simulink model "Test"  (R2018a)
settings: Solver=VariableStepAuto  StartTime=0.0  StopTime=1  RelTol=1e-3
libraries: powerlib x37, dspstat3 x1
settings Model: Creator=AL-MOSTAFA  LastModifiedBy=AL-MOSTAFA

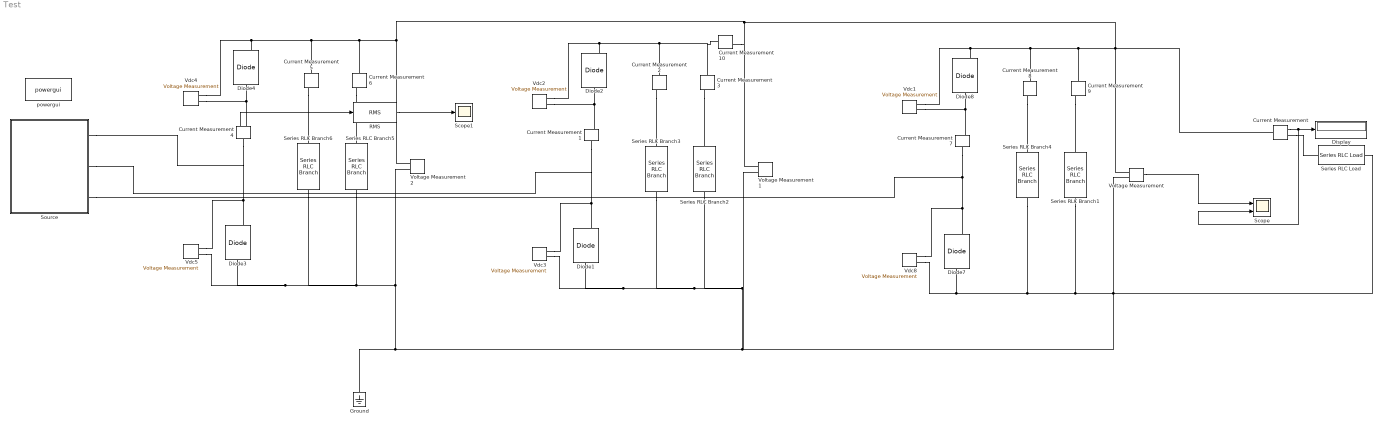
== system Test ==
  Current Measurement{,1..9} (10 alike) : powerlib/Measurements/Current Measurement  PhasorSimulation=off  OutputType=Complex  PSBequivalent=0
  Current Measurement10 : powerlib/Measurements/Current Measurement  PhasorSimulation=off  OutputType=Magnitude  PSBequivalent=0
  Diode{1..4,7..8} (6 alike) : powerlib/Power Electronics/Diode  Ron=0.001  Lon=0  Vf=0.8  IC=0  UseSnubber=0  Rs=500  Cs=250e-9  Measurements=on
  Display : Display
  Ground : powerlib/Elements/Ground  LConnTagsString=a
  RMS : dspstat3/RMS  run=off  directionMode=Each column  dimension=1  InputProcessing=Columns as channels (frame based)  reset_popup=None
  Scope : Scope  NumInputPorts=2
  Scope1 : Scope
  Series RLC Branch{1..6} (6 alike) : powerlib/Elements/Series RLC Branch  LConnTagsString=__new0  RConnTagsString=__new0  BranchType=C  Resistance=10  Inductance=1e-3  SetiL0=off  InitialCurrent=0  Capacitance=500*10^-6  Setx0=off  InitialVoltage=0  Measurements=None
  Series RLC Load : powerlib/Elements/Series RLC Load  LConnTagsString=a  RConnTagsString=__new0  NominalVoltage=500  NominalFrequency=60  ActivePower=5e3  InductivePower=0  CapacitivePower=0  Setx0=off  InitialVoltage=0  SetiL0=off  InitialCurrent=0  Measurements=None  LoadType=constant Z
  Source : Subsystem
  Vdc{1..5,8} (6 alike) : powerlib/Measurements/Voltage Measurement  PhasorSimulation=off  OutputType=Complex  PSBequivalent=0
  Voltage Measurement : powerlib/Measurements/Voltage Measurement  PhasorSimulation=off  OutputType=Complex  PSBequivalent=0
  Voltage Measurement1 : powerlib/Measurements/Voltage Measurement  PhasorSimulation=off  OutputType=Complex  PSBequivalent=0
  Voltage Measurement2 : powerlib/Measurements/Voltage Measurement  PhasorSimulation=off  OutputType=Complex  PSBequivalent=0
  powergui : powerlib/powergui  Priority=1  SimulationMode=Continuous  SampleTime=50e-6  frequency=60  Iterations=50  frequencyindice=50  Pbase=100e6  ErrMax=1e-4  UnitsV=kV  UnitsW=MW  buscounter=0  FunctionMessages=off  echomessages=off  EnableUseOfTLC=off  CurrentSourceSwitches=off  DisableSnubberDevices=off  DisableRonSwitches=off  DisableVfSwitches=off  DisplayEquations=off  SolverType=Tustin/Backward Euler (TBE)  Interpol=off  ExternalGateDelay=off  methode=off  Ts=100  x0status=blocks  SPID=on  SwTol=0  HookPort=off  RestoreLinks=warning  ResistiveCurrentMeasurement=off  Frange=[0:2:500]  Ylog=off  Xlog=on  ShowGrid=off  save=off  variable=ZData  structure=0  ZoomFFT=off  StartTime=0.0  cycles=1  DisplayStyle=1  fundamental=60  FreqAxis=off  MaxFrequency=1000  frequencyindicesteady=1  RmsSteady=1  display=off
  wires:
  Current Measurement/1 -> Scope/2, Display/1
  Current Measurement4/1 -> RMS/1
  Voltage Measurement/1 -> Scope/1
  RMS/1 -> Scope1/1
  connections:
  Current Measurement/RConn1 -- Series RLC Load/LConn1
  Current Measurement7/RConn1 -- Diode8/LConn1 -- Vdc1/LConn1
  Series RLC Branch1/RConn1 -- Series RLC Load/RConn1 -- Series RLC Branch2/RConn1 -- Series RLC Branch3/RConn1 -- Vdc3/LConn1 -- Diode1/LConn1 -- Voltage Measurement1/LConn2 -- Ground/LConn1 -- Diode3/LConn1 -- Vdc5/LConn1 -- Series RLC Branch6/RConn1 -- Series RLC Branch5/RConn1 -- Voltage Measurement2/LConn2 -- Voltage Measurement/LConn2 -- Series RLC Branch4/RConn1 -- Vdc8/LConn1 -- Diode7/LConn1
  Current Measurement7/LConn1 -- Source/RConn3 -- Diode7/RConn1 -- Vdc8/LConn2
  Vdc3/LConn2 -- Source/RConn2 -- Current Measurement1/LConn1 -- Diode1/RConn1
  Vdc5/LConn2 -- Source/RConn1 -- Current Measurement4/LConn1 -- Diode3/RConn1
  Current Measurement4/RConn1 -- Diode4/LConn1 -- Vdc4/LConn1
  Voltage Measurement/LConn1 -- Current Measurement/LConn1 -- Current Measurement10/RConn1 -- Voltage Measurement1/LConn1 -- Voltage Measurement2/LConn1 -- Current Measurement6/LConn1 -- Diode4/RConn1 -- Vdc4/LConn2 -- Current Measurement5/LConn1 -- Current Measurement9/LConn1 -- Current Measurement8/LConn1 -- Vdc1/LConn2 -- Diode8/RConn1
  Current Measurement1/RConn1 -- Diode2/LConn1 -- Vdc2/LConn1
  Current Measurement9/RConn1 -- Series RLC Branch1/LConn1
  Current Measurement5/RConn1 -- Series RLC Branch6/LConn1
  Current Measurement8/RConn1 -- Series RLC Branch4/LConn1
  Current Measurement2/RConn1 -- Series RLC Branch3/LConn1
  Current Measurement3/RConn1 -- Series RLC Branch2/LConn1
  Current Measurement6/RConn1 -- Series RLC Branch5/LConn1
  Current Measurement2/LConn1 -- Current Measurement10/LConn1 -- Current Measurement3/LConn1 -- Diode2/RConn1 -- Vdc2/LConn2

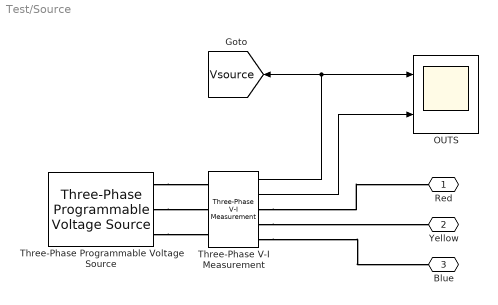
== system Test/Source ==
  OUTS : Scope  NumInputPorts=2
  Three-Phase Programmable Voltage Source : powerlib/Electrical Sources/Three-Phase Programmable Voltage Source  PositiveSequence="[380  0 50]"  VariationEntity=None  VariationType=Table of time-amplitude pairs  VariationTypeAlt=Step  VariationStep=0.5  VariationRate=10  VariationMagnitude=0.3  VariationFrequency=2  VariationTiming=[1 2]  VariationPhaseA=off  Amplitudes=[1 0.8 1.2 1.0]  TimeValues=[0 0.1 0.15 0.2]  HarmonicGeneration=off  HarmonicA=[3 0.2 -25 0]  HarmonicB=[2 0.15 35 2]  Timing="[0.05  3]"  BusType=swing  Pref=0  Qref=0  Qmin=-inf  Qmax=inf
  Three-Phase V-I Measurement : powerlib/Measurements/Three-Phase V-I Measurement  VoltageMeasurement=phase-to-ground  SetLabelV=off  LabelV=Vabc  Vpu=off  VpuLL=off  CurrentMeasurement=yes  SetLabelI=off  LabelI=Iabc  Ipu=off  Pbase=100e6  Vbase=500e3  OutputType=Complex  PhasorSimulation=off  PSBequivalent=0
  Red : PMIOPort  Side=Right
  Yellow : PMIOPort  Port=2  Side=Right
  Blue : PMIOPort  Port=3  Side=Right
  tag scope: Vsource=global
  wires:
  Three-Phase V-I Measurement/1 -> [Vsource], OUTS/1
  Three-Phase V-I Measurement/2 -> OUTS/2
  connections:
  Three-Phase V-I Measurement/RConn3 -- Blue/RConn1
  Three-Phase V-I Measurement/RConn1 -- Red/RConn1
  Three-Phase V-I Measurement/RConn2 -- Yellow/RConn1
  Three-Phase Programmable Voltage Source/RConn1 -- Three-Phase V-I Measurement/LConn1
  Three-Phase Programmable Voltage Source/RConn2 -- Three-Phase V-I Measurement/LConn2
  Three-Phase Programmable Voltage Source/RConn3 -- Three-Phase V-I Measurement/LConn3
